simulink model "PIDv0"  (R2022a)
settings: Solver=VariableStepAuto  StartTime=0.0  StopTime=10.0  RelTol=1e-3
undefined symbols (not defined in the file): Kd, Ki, Kp
settings Model: Creator=leonj  LastModifiedBy=leonj

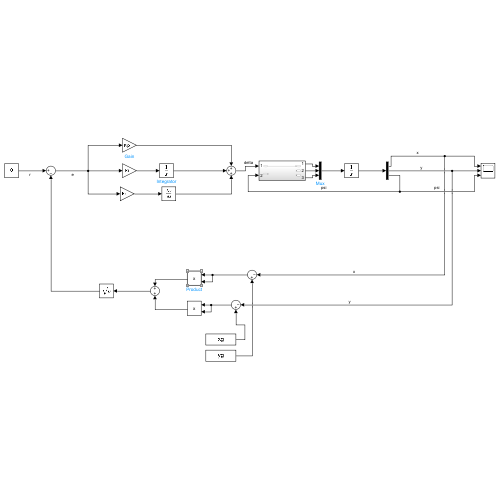
[thumbnail: Simulink's stored preview of the top-level diagram]
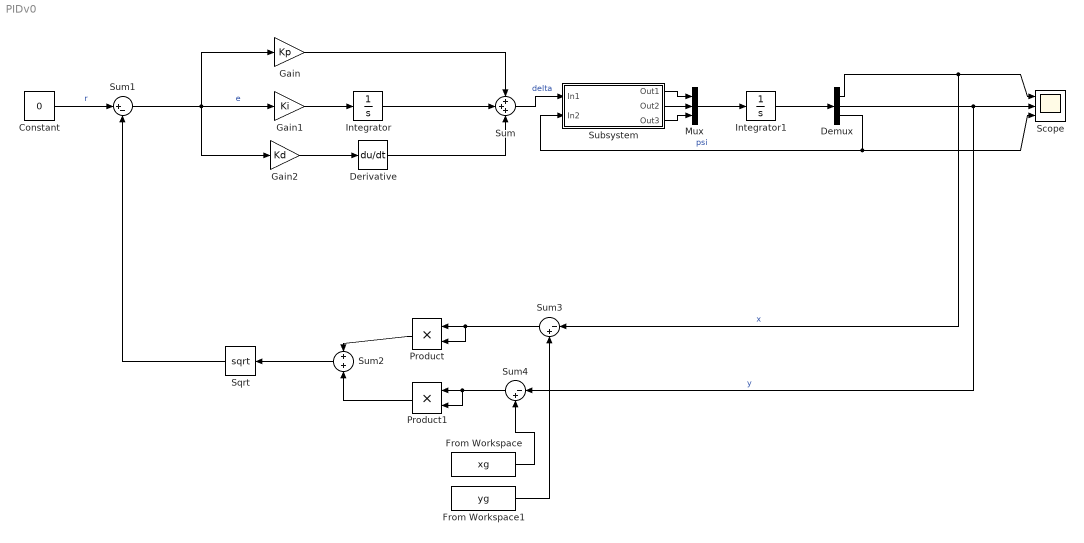
== system PIDv0 ==
  Constant : Constant  Value=0
  Demux : Demux  Outputs=3
  Derivative : Derivative
  From Workspace : FromWorkspace  VariableName=xg
  From Workspace1 : FromWorkspace  VariableName=yg
  Gain : Gain  Gain=Kp
  Gain1 : Gain  Gain=Ki
  Gain2 : Gain  Gain=Kd
  Integrator : Integrator
  Integrator1 : Integrator
  Mux : Mux  Inputs=3
  Product : Product
  Product1 : Product
  Scope : Scope  NumInputPorts=3
  Sqrt : Sqrt
  Subsystem : Subsystem
  Sum : Sum  Inputs=+++
  Sum1 : Sum  Inputs=|+-
  Sum2 : Sum  Inputs=+|+
  Sum3 : Sum  Inputs=|-+
  Sum4 : Sum  Inputs=|-+
  wires:
  Constant/1 -> Sum1/1  "r"
  Gain2/1 -> Derivative/1
  Gain1/1 -> Integrator/1
  Integrator/1 -> Sum/2
  Gain/1 -> Sum/1
  Derivative/1 -> Sum/3
  Sum1/1 -> Gain/1, Gain1/1, Gain2/1  "e"
  Sum/1 -> Subsystem/1(In1)  "delta"
  Sum2/1 -> Sqrt/1
  Product/1 -> Sum2/1
  Product1/1 -> Sum2/2
  Sqrt/1 -> Sum1/2
  Integrator1/1 -> Demux/1
  Demux/3 -> Subsystem/2(In2), Scope/3  "psi"
  Subsystem/3(Out3) -> Mux/3
  Subsystem/2(Out2) -> Mux/2
  Subsystem/1(Out1) -> Mux/1
  Mux/1 -> Integrator1/1
  Demux/2 -> Sum4/1, Scope/2  "y"
  Demux/1 -> Sum3/1, Scope/1  "x"
  Sum3/1 -> Product/2, Product/1
  Sum4/1 -> Product1/2, Product1/1
  From Workspace/1 -> Sum4/2
  From Workspace1/1 -> Sum3/2

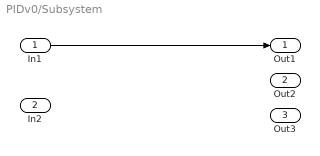
== system PIDv0/Subsystem ==
  In1 : Inport
  In2 : Inport  Port=2
  Out1 : Outport
  Out2 : Outport  Port=2
  Out3 : Outport  Port=3
  wires:
  In1/1 -> Out1/1
